simulink model "Traffic_Light_Stateflow"  (R2016b)
settings: Solver=FixedStepDiscrete  StartTime=0.0  StopTime=inf  FixedStep=0.1  RelTol=1e-3  EnableMultiTasking=on
settings Model: Creator=Saher Ghanem  LastModifiedBy=Saher Ghanem
settings SolverCC: AutoInsertRateTranBlk=on
settings DataIOCC: LimitDataPoints=on
settings OptimizationCC: LifeSpan=inf
settings DebuggingCC: AllowSymbolicDim=off  SFUnexpectedBacktrackingDiag=warning  SFNoUnconditionalDefaultTransitionDiag=warning  SFExecutionAtInitializationDiag=none
settings GRTTargetCC: TargetLangStandard=C89/C90 (ANSI)  GeneratePreprocessorConditionals=Disable all
settings ConfigComp: CovMetricSettings=dw  CovHtmlReporting=on  CovSaveCumulativeToWorkspaceVar=on  CovSaveSingleToWorkspaceVar=on  CovExternalEMLEnable=off  CovSFcnEnable=off

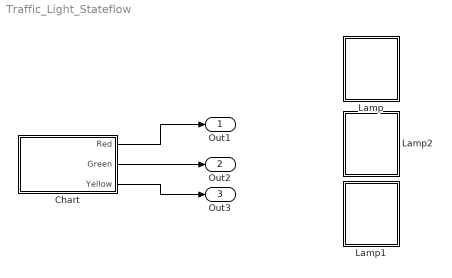
== system Traffic_Light_Stateflow ==
  Chart : Stateflow chart  TreatAsAtomicUnit=on
  Lamp : Subsystem  DialogController=hmiCreateDDGDialog  IsWebBlock=on  mask(MWDashboardBlock){webBlockId=05349115-8cda-4797-8c96-c1f07842b1ba, webBlockType=lamp, ShowInLibBrowser=on, ShowInitialText=on, HMISrcModelName=Traffic_Light_Stateflow}
      mask prompts: webBlockType "WebBlock Type"; HMISrcModelName "Source Model"
      mask help: SimulinkHMI:dialogs:LampDialogDesc
      mask Help: helpview([docroot '/mapfiles/simulink.map'], 'hmi_lamp')
      mask Display:
      | if strcmp(get_param(bdroot(gcb),'BlockDiagramType'), 'library')
      |     image([(matlabroot) '/toolbox/simulink/hmi/icons/Lamp.png']);
      | end
  Lamp1 : Subsystem  DialogController=hmiCreateDDGDialog  IsWebBlock=on  mask(MWDashboardBlock){webBlockId=622d8122-ec2b-4326-bbee-5d3c525d0309, webBlockType=lamp, ShowInLibBrowser=on, ShowInitialText=on, HMISrcModelName=Traffic_Light_Stateflow}
      mask prompts: webBlockType "WebBlock Type"; HMISrcModelName "Source Model"
      mask help: SimulinkHMI:dialogs:LampDialogDesc
      mask Help: helpview([docroot '/mapfiles/simulink.map'], 'hmi_lamp')
      mask Display:
      | if strcmp(get_param(bdroot(gcb),'BlockDiagramType'), 'library')
      |     image([(matlabroot) '/toolbox/simulink/hmi/icons/Lamp.png']);
      | end
  Lamp2 : Subsystem  DialogController=hmiCreateDDGDialog  IsWebBlock=on  mask(MWDashboardBlock){webBlockId=16a29903-56e2-44fa-8dc1-2b1dbdf39ad4, webBlockType=lamp, ShowInLibBrowser=on, ShowInitialText=on, HMISrcModelName=Traffic_Light_Stateflow}
      mask prompts: webBlockType "WebBlock Type"; HMISrcModelName "Source Model"
      mask help: SimulinkHMI:dialogs:LampDialogDesc
      mask Help: helpview([docroot '/mapfiles/simulink.map'], 'hmi_lamp')
      mask Display:
      | if strcmp(get_param(bdroot(gcb),'BlockDiagramType'), 'library')
      |     image([(matlabroot) '/toolbox/simulink/hmi/icons/Lamp.png']);
      | end
  Out1 : Outport
  Out2 : Outport  Port=2
  Out3 : Outport  Port=3
  wires:
  Chart/2(Green) -> Out2/1
  Chart/1(Red) -> Out1/1
  Chart/3(Yellow) -> Out3/1

== system Traffic_Light_Stateflow/Lamp ==

== system Traffic_Light_Stateflow/Lamp1 ==

== system Traffic_Light_Stateflow/Lamp2 ==

== stateflow chart Traffic_Light_Stateflow/Chart ==
  state Yellow_Dark
    entry:
    Red=0;
    Green=0;
    Yellow=1;
  state Red_Light
    entry:
    Red=1;
    Green=0;
    Yellow=0;
  state Green_Light1
    entry:
    Red=0;
    Green=1;
    Yellow=0;
  (default) -> Red_Light
  Yellow_Dark -> Green_Light1 : after(1000,tick)
  Red_Light -> Yellow_Dark : after(1000,tick)
  Green_Light1 -> Red_Light : after(1000,tick)
  data: Red output; Green output; Yellow output
